simulink model "dezim_1"  (Simulink 7.8)
settings: Solver=ode45  StartTime=0.0  StopTime=1  RelTol=1e-3
undefined symbols (not defined in the file or in its folder): get
libraries: dspsigops x2, dspsnks4 x2, dsparch4 x1
settings Model: Creator=svenhoffmann  LastModifiedBy=josef  ExtModeAutoUpdateStatusClock=off
settings DataIOCC: SignalLoggingName=sigsOut
settings OptimizationCC: InitFltsAndDblsToZero=on
settings DebuggingCC: SaveWithParameterizedLinksMsg=none  SignalResolutionControl=TryResolveAllWithWarning  SolverPrmCheckMsg=none  MultiTaskDSMMsg=warning  MultiTaskCondExecSysMsg=none  FcnCallInpInsideContextMsg=Use local settings  StrictBusMsg=None
settings HardwareCC: TargetUnknown=on
settings RTWCC: IncludeERTFirstTime=on
settings GRTTargetCC: TargetFcnLib=ansi_tfl_tmw.mat

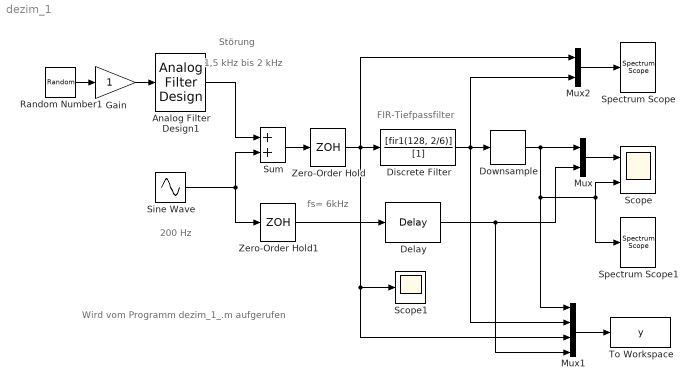
== system dezim_1 ==
  note: Störung
  note: 200 Hz
  note: 1,5 kHz bis
      | 2 kHz
  note: fs=
      | 6kHz
  note: FIR-Tiefpassfilter
  note: Wird vom Programm dezim_1_.m
      | aufgerufen
  Analog Filter Design1 : dsparch4/Analog Filter Design  method=Butterworth  filttype=Bandpass  N=8  Wlo=2*pi*1500  Whi=2*pi*2000  Rp=2  Rs=40
  Delay : dspsigops/Delay  InputProcessing=Inherited (this choice will be removed - see release notes)  dly_unit=Samples  delay=64  ic_detail=off  dif_ic_for_ch=off  dif_ic_for_dly=off  ic=0  reset_popup=None
  Discrete Filter : DiscreteFilter  Numerator=[fir1(128, 2/6)]  Denominator=[1]  SampleTime=1/6000
  Downsample : dspsigops/Downsample  N=3  phase=0  InputProcessing=Inherited (this choice will be removed - see release notes)  RateOptions=Enforce single-rate processing  smode=Allow multirate  fmode=Maintain input frame size  ic=0
  Gain : Gain  SaturateOnIntegerOverflow=on  OutDataTypeStr=Inherit: Same as input  ParamDataTypeStr=Inherit: Same as input
  Mux : Mux  Inputs=2
  Mux1 : Mux
  Mux2 : Mux  Inputs=2
  Random Number1 : RandomNumber  Seed=1739  SampleTime=0
  Scope : Scope  NumInputPorts=2
      settings: YMin=-1.2~-5  YMax=1.1~5
  Scope1 : Scope
  Sine Wave : Sin  Frequency=2*pi*200  SampleTime=0
  Spectrum Scope : dspsnks4/Spectrum Scope  ScopeProperties=on  Domain=Frequency  HorizSpan=1  UseBuffer=on  BufferSize=256  Overlap=64  TreatMby1Signals=M channels  inpFftLenInherit=off  FFTlength=128  numAvg=10  DisplayProperties=off  AxisGrid=on  Memory=off  FrameNumber=on  AxisLegend=off  AxisZoom=off  OpenScopeAtSimStart=on  OpenScopeImmediately=off  FigPos=get(0,'defaultfigureposition')  AxisProperties=off  XUnits=Hertz  XRange=[0...Fs]  XDisplay=0  InheritXIncr=off  XIncr=1/6000  XLabel=Samples  XLimit=Auto  YUnits=dBW/Hertz  XMax=1  XMin=0  YLabel=Magnitude, dB  LineProperties=off  wintypeSpecScope=Hann  RsSpecScope=50  betaSpecScope=5  winsampSpecScope=Periodic  XAxisParamsVer=6.8  isFrameUpgraded=on
      settings: YMin=-179.4872  YMax=-20.7008
  Spectrum Scope1 : dspsnks4/Spectrum Scope  ScopeProperties=off  Domain=Frequency  HorizSpan=1  UseBuffer=on  BufferSize=256  Overlap=64  TreatMby1Signals=M channels  inpFftLenInherit=off  FFTlength=128  numAvg=10  DisplayProperties=off  AxisGrid=on  Memory=off  FrameNumber=on  AxisLegend=off  AxisZoom=off  OpenScopeAtSimStart=on  OpenScopeImmediately=off  FigPos=get(0,'defaultfigureposition')  AxisProperties=on  XUnits=Hertz  XRange=[0...Fs]  XDisplay=0  InheritXIncr=off  XIncr=1/2000  XLabel=Samples  XLimit=Auto  YUnits=dBW/Hertz  XMax=1  XMin=0  YLabel=Magnitude, dB  LineProperties=off  wintypeSpecScope=Hann  RsSpecScope=50  betaSpecScope=5  winsampSpecScope=Periodic  XAxisParamsVer=6.8  isFrameUpgraded=on
      settings: YMin=-99.1635  YMax=-16.9836
  Sum : Sum  SaturateOnIntegerOverflow=on
  To Workspace : ToWorkspace  VariableName=y  SampleTime=-1  SaveFormat=Structure With Time
  Zero-Order Hold : ZeroOrderHold  SampleTime=1/6000
  Zero-Order Hold1 : ZeroOrderHold  SampleTime=1/6000
  wires:
  Random Number1/1 -> Gain/1
  Sine Wave/1 -> Sum/2, Zero-Order Hold1/1
  Gain/1 -> Analog Filter Design1/1
  Analog Filter Design1/1 -> Sum/1
  Sum/1 -> Zero-Order Hold/1
  Zero-Order Hold/1 -> Discrete Filter/1, Mux2/1, Scope1/1, Mux1/3
  Discrete Filter/1 -> Downsample/1, Mux2/2, Mux1/2
  Downsample/1 -> Mux/1, Mux1/1, Scope/2, Spectrum Scope1/1
  Mux/1 -> Scope/1
  Delay/1 -> Mux/2, Mux1/4
  Zero-Order Hold1/1 -> Delay/1
  Mux1/1 -> To Workspace/1
  Mux2/1 -> Spectrum Scope/1
